simulink model "prova_librerie_arduino"  (R2024b)
settings: Solver=FixedStepAuto  StartTime=0.0  StopTime=10.0  RelTol=1e-3  EnableMultiTasking=on
libraries: arduinolib x2
settings Model: ExtModeTrigDuration=2  Creator=Andrea Blumer  LastModifiedBy=Andrea Blumer
settings SolverCC: AutoInsertRateTranBlk=on
settings OptimizationCC: EnhancedBackFolding=on  PassReuseOutputArgsAs=Individual arguments  ZeroExternalMemoryAtStartup=off  ZeroInternalMemoryAtStartup=off  MaxStackSize=64  OptimizeBlockOrder=speed  DifferentSizesBufferReuse=on  OptimizationCustomize=off  EfficientTunableParamExpr=on
settings DebuggingCC: ParameterTunabilityLossMsg=error
settings HardwareCC: ProdBitPerInt=16  ProdBitPerPointer=16  ProdBitPerSizeT=16  ProdBitPerPtrDiffT=16  ProdLargestAtomicFloat=None  ProdWordSize=8  ProdHWDeviceType=Atmel->AVR
settings SFSimCC: MATLABDynamicMemAlloc=off
settings RTWCC: Description=Embedded Coder  SystemTargetFile=ert.tlc  HardwareBoard=Arduino Mega 2560  TemplateMakefile=ert_default_tmf  Toolchain=Arduino AVR  BuildConfiguration=Faster Runs
settings CodeAppCC: ForceParamTrailComments=on  IgnoreCustomStorageClasses=off  OperatorAnnotations=on  SimulinkDataObjDesc=on  SFDataObjDesc=on  InsertBlockDesc=on
settings ERTTargetCC: SupportContinuousTime=on  SupportVariableSizeSignals=on  ExtModeTransport=3  ExtModeStaticAlloc=on  ExtModeAutomaticAllocSize=off  ExtModeStaticAllocSize=2048  ExtModeMexFile=ext_xcp  ExtModeIntrfLevel=Level2 - Open  InlinedParameterPlacement=Hierarchical

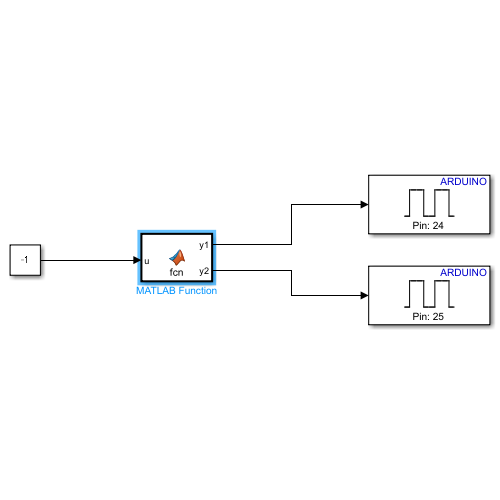
[thumbnail: Simulink's stored preview of the top-level diagram]
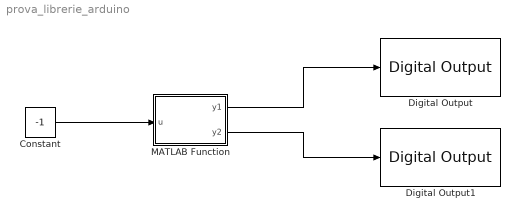
== system prova_librerie_arduino ==
  Constant : Constant  Value=-1
  Digital Output : arduinolib/Digital Output  pinNumber=24  Direction=output  blockPlatform=arduino
      settings: SourceProductName=Common
  Digital Output1 : arduinolib/Digital Output  pinNumber=25  Direction=output  blockPlatform=arduino
      settings: SourceProductName=Common
  MATLAB Function : MATLAB Function  TreatAsAtomicUnit=on
  wires:
  MATLAB Function/1(y1) -> Digital Output/1
  MATLAB Function/2(y2) -> Digital Output1/1
  Constant/1 -> MATLAB Function/1(u)

== matlab function prova_librerie_arduino/MATLAB Function ==
  data: u input; y1 output; y2 output
function [y1, y2] = fcn(u)
if u > 0
    y1 = 1;
    y2 = 0;
else
    y1 = 1;
    y2 = 1;
end
return
